simulink subsystem "processor"  (R2025b)
settings: Solver=VariableStepAuto  StartTime=0.0  StopTime=10.0  RelTol=1e-3
undefined symbols (not defined in the file): samplingrate
libraries: simulink x2
settings Model: Creator=finnb  LastModifiedBy=finnb

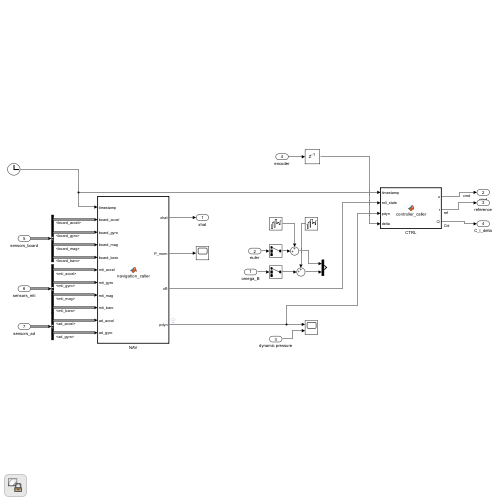
[thumbnail: Simulink's stored preview of the top-level diagram]
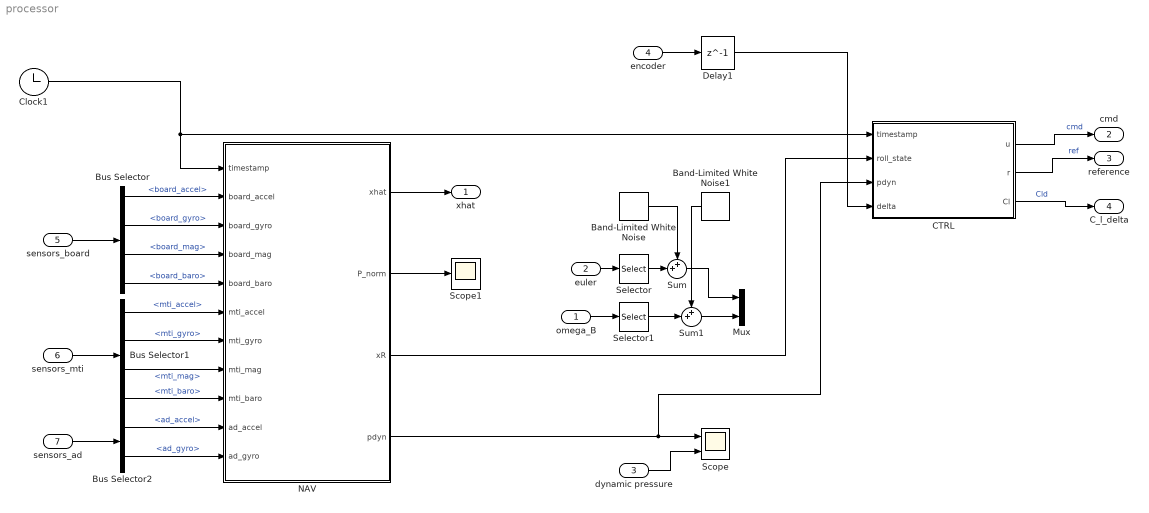
== system processor ==
  omega_B : Inport
  euler : Inport  Port=2
  dynamic pressure : Inport  Port=3
  encoder : Inport  Port=4
  sensors_board : Inport  Port=5
  sensors_mti : Inport  Port=6
  sensors_ad : Inport  Port=7
  Band-Limited White Noise : simulink/Sources/Band-Limited White Noise  Cov=2e-10  Ts=0.1  seed=[233256]
  Band-Limited White Noise1 : simulink/Sources/Band-Limited White Noise  Cov=2e-8  Ts=samplingrate  seed=[2345]
  Bus Selector : BusSelector  OutputSignals=board_accel,board_gyro,board_mag,board_baro
  Bus Selector1 : BusSelector  OutputSignals=mti_accel,mti_gyro,mti_mag,mti_baro
  Bus Selector2 : BusSelector  OutputSignals=ad_accel,ad_gyro
  CTRL : MATLAB Function  TreatAsAtomicUnit=on
  Clock1 : Clock
  Delay1 : Delay  DelayLength=1
  Mux : Mux  Inputs=2
  NAV : MATLAB Function  TreatAsAtomicUnit=on
  Scope : Scope  NumInputPorts=2
      settings: ActiveDisplayYMinimum=-5455.3887488403561  ActiveDisplayYMaximum=7906.9461618994392  DataLoggingVariableName=ScopeData19
  Scope1 : Scope
      settings: ActiveDisplayYMinimum=-0.025666300383096634  ActiveDisplayYMaximum=0.23099670344786977  DataLoggingVariableName=ScopeData2
  Selector : Selector  InputPortWidth=3  IndexOptions=Index vector (dialog)  Indices=[1]  OutputSizes=1
  Selector1 : Selector  InputPortWidth=3  IndexOptions=Index vector (dialog)  Indices=[1]  OutputSizes=1
  Sum : Sum  Inputs=++|
  Sum1 : Sum  Inputs=++|
  xhat : Outport
  cmd : Outport  Port=2
  reference : Outport  Port=3
  C_l_delta : Outport  Port=4
  wires:
  Clock1/1 -> CTRL/1(timestamp), NAV/1(timestamp)
  NAV/1(xhat) -> xhat/1
  encoder/1 -> Delay1/1
  CTRL/2(r) -> reference/1  "ref"
  CTRL/1(u) -> cmd/1  "cmd"
  Delay1/1 -> CTRL/4(delta)
  NAV/3(xR) -> CTRL/2(roll_state)
  Selector/1 -> Sum/2
  Selector1/1 -> Sum1/2
  euler/1 -> Selector/1
  omega_B/1 -> Selector1/1
  NAV/4(pdyn) -> CTRL/3(pdyn), Scope/1
  CTRL/3(Cl) -> C_l_delta/1  "Cld"
  Sum/1 -> Mux/1
  Band-Limited White Noise/1 -> Sum/1
  Sum1/1 -> Mux/2
  Band-Limited White Noise1/1 -> Sum1/1
  sensors_board/1 -> Bus Selector/1
  sensors_mti/1 -> Bus Selector1/1
  sensors_ad/1 -> Bus Selector2/1
  Bus Selector/1 -> NAV/2(board_accel)  "<board_accel>"
  Bus Selector/2 -> NAV/3(board_gyro)  "<board_gyro>"
  Bus Selector/3 -> NAV/4(board_mag)  "<board_mag>"
  Bus Selector/4 -> NAV/5(board_baro)  "<board_baro>"
  Bus Selector1/1 -> NAV/6(mti_accel)  "<mti_accel>"
  Bus Selector1/2 -> NAV/7(mti_gyro)  "<mti_gyro>"
  Bus Selector1/3 -> NAV/8(mti_mag)  "<mti_mag>"
  Bus Selector1/4 -> NAV/9(mti_baro)  "<mti_baro>"
  Bus Selector2/2 -> NAV/11(ad_gyro)  "<ad_gyro>"
  Bus Selector2/1 -> NAV/10(ad_accel)  "<ad_accel>"
  NAV/2(P_norm) -> Scope1/1
  dynamic pressure/1 -> Scope/2

== matlab function processor/CTRL ==
  settings: updateMethod=DISCRETE  sampleTime=samplingrate
  data: timestamp input size=1; roll_state input size=2; pdyn input size=1; delta input size=1; u output size=1; r output size=1; Cl output size=1
function [u, r, Cl] = controller_caller(timestamp,roll_state, pdyn, delta)
    [u, r, Cl] = controller_module(timestamp, roll_state, pdyn, delta);
end

== matlab function processor/NAV ==
  settings: updateMethod=DISCRETE  sampleTime=samplingrate
  data: timestamp input size=1; xhat output; P_norm output; xR output; board_accel input Bus: Sensor3DBus; board_gyro input Bus: Sensor3DBus; board_mag input Bus: Sensor3DBus; pdyn output; board_baro input Bus: Sensor1DBus; mti_accel input Bus: Sensor3DBus; mti_gyro input Bus: Sensor3DBus; mti_mag input Bus: Sensor3DBus; mti_baro input Bus: Sensor1DBus; ad_accel input Bus: Sensor3DBus; ad_gyro input Bus: Sensor3DBus
function [xhat, P_norm, xR, pdyn] = navigation_caller(timestamp, board_accel, board_gyro, board_mag, board_baro, mti_accel, mti_gyro, mti_mag, mti_baro, ad_accel, ad_gyro)
    %#codegen

    %% IMU handler mock (rotation correction)
    board_accel.meas = imu_handler(board_accel.meas, "board");
    board_gyro.meas = imu_handler(board_gyro.meas, "board");
    mti_accel.meas = imu_handler(mti_accel.meas, "mti");
    mti_gyro.meas = imu_handler(mti_gyro.meas, "mti");
    ad_accel.meas = imu_handler(ad_accel.meas, "ad");
    ad_gyro.meas = imu_handler(ad_gyro.meas, "ad");
    %%% mag and baro do not need to be rotation corrected    
   
    
    %% Navigation
    xhat = zeros(11,1);         
    P_norm = 0;
    xR = zeros(2,1);
    pdyn = 0;

    [xhat, P_norm, airdata, xR] = navigation_module(timestamp, board_accel, board_gyro, mti_accel, mti_gyro, ad_accel, ad_gyro, board_baro, board_mag, mti_baro, mti_mag);
    pdyn = airdata.dynamic_pressure;    
end
